simulink model "HevMmPowertrainController"  (R2020a)
settings: Solver=ode4  StartTime=0.0  StopTime=inf  FixedStep=.01  RelTol=1e-3  EnableMultiTasking=on
model workspace (MAT data in the model file):
  ChrgSOCHi = 80
  ChrgSOCLo = 70
  EngCltchOffTractiveForce = 3000
  EngCltchOffVehSpd = 70
  EngCltchOnTractiveForce = 2000
  EngCltchOnVehSpd = 80
  EngCltchOnWait = 5
  EngDriveRatio = 0.813008130081
  FricBrakeCmd = [0 0 12 24 36 48 60]
  FricBrakeCmdBpt = [0 0.1 0.2 0.4 0.6 0.8 1]
  MaxChrgPwr = 50000
  MaxRegenPwr = 10000
  MotGbRatio = 2.45
  Ndiff = 3.421
  Rm = 0.17778
  Ts = 0.01
  disk_abore = 0.05
  eng.pwr = [15052.6315789 19736.8421053 24421.0526316 29105.2631579 33789.4736842 38473.6842105 43157.8947368 47842.1052632 52526.3157895 57210.5263158 61894.7368421 66578.9473684 71263.1578947 75947.3684211 80631.5789474 85315.7894737 90000]
  eng.spd = [1448.84862461 1712.99052669 1980.33600187 2249.1155588 2517.55970613 2783.89895252 3046.3638066 3303.18477703 3552.59237246 3792.81710154 4022.08947291 4238.63999523 4440.69917715 4626.49752731 4794.26555436 4942.23376695 5068.63267374]
  eng.bsfc = [256.743221884 250.98807985 246.162934447 242.291845325 239.398872138 237.508074537 236.643512177 236.829244708 238.089331783 240.447833055 243.928808176 248.556316798 254.354418575 261.347173158 269.5586402 279.012879353 289.73395027]
  eng.trq = [99.2112225513 110.02568665 117.759751017 123.57514891 128.166058939 131.971967205 135.285068696 138.308475993 141.18967656 144.040766791 146.951280713 149.9967243 153.244568751 156.75874496 160.603298419 164.845657961 169.559869104]
  eng.idle = 1448.84862461
  eng.ff = [0.00107351698039 0.00137603113953 0.00166987721613 0.00195887997755 0.00224698941392 0.00253828073811 0.00283695438574 0.00314733601519 0.00347387650759 0.00382115196682 0.00419386371951 0.00459683831506 0.00503502752559 0.005513508346 0.00603748299394 0.00661227890981 0.00724334875674]
  eng.pwrin = [46556.889434 59676.4939829 72420.1762428 84953.8108807 97448.7032942 110081.589612 123034.636693 136495.442128 150657.034239 165717.872078 181881.845427 199358.274801 218361.911444 239112.937333 261836.965174 286765.038405 314133.631195]
  gen.max_trq = 247.580645161
  gen.max_pwr = 102.101761242
  gen.spd = [0 500 1000 1500 2000 2500 3000 3500 3938.11074919 4000 4500 5000 5500 6000 6500 7000 7500 8000 8500 9000 9500 10000 10500 11000 11500 12000 12500]
  gen.trq = [247.580645161 247.580645161 247.580645161 247.580645161 247.580645161 247.580645161 247.580645161 247.580645161 247.580645161 243.75 216.666666667 195 177.272727273 162.5 150 139.285714286 130 121.875 114.705882353 108.333333333 102.631578947 97.5 92.8571428571 88.6363636364 84.7826086957 81.25 78]
  gen.trq_cp = [243.75 216.666666667 195 177.272727273 162.5 150 139.285714286 130 121.875 114.705882353 108.333333333 102.631578947 97.5 92.8571428571 88.6363636364 84.7826086957 81.25 78]
  gen.J = 0.02
  gen.damp = 0.001
  gen.Tc = 0.02
  gen.map.spdindex = [0 1000 2000 3000 3857 4000 5000 6000 7000 8000 9000 10000 11000 12000 12584]
  gen.map.trqindex = [10 25 50 75 100 125 150 175 200 225 235.201612903]
  gen.map.eff = [84  90  90  90  90  90  90  90  90  90  90  90  90  90  90; 84  90  93  95  95  95  96  95  95  95  95  93  93  93  93; 84  90  93  95  95  95  96  95  96  95  95  95  95  93  93; 84  90  93  95  95  95  96  96  96  95  95  93  95  93  93; 84  90  93  95  95  95  96  96  96  95  95  93  93  93  93; 84  88  90  93  93  95  95  96  95  93  93  93  93  93  93; 84  88  90  90  90  93  95  95  93  93  93  93  93  93  93; 84  88  90  90  90  90  93  93  93  93  93  93  93  93  93; 84  84  88  90  90  90  90  93  93  93  93  93  93  93  93; 84  84  88  90  90  90  90  93  93  93  93  93  93  93  93; 84  84  88  90  90  90  90  93  93  93  93  93  93  93  93]
  gen.m = 20
  gen.Cp = 200
  mot.max_trq = 307
  mot.max_pwr = 124
  mot.spd = [0 500 1000 1500 2000 2500 3000 3500 3857.04487493 4000 4500 5000 5500 6000 6500 7000 7500 8000 8500 9000 9500 10000 10500 11000 11500 12000 12500]
  mot.trq = [307 307 307 307 307 307 307 307 307 296.028194151 263.136172579 236.822555321 215.29323211 197.352129434 182.171196401 169.158968086 157.881703547 148.014097075 139.307385483 131.568086289 124.643450169 118.41127766 112.772645391 107.646616055 102.9663284 98.676064717 94.7290221283]
  mot.trq_cp = [296.028194151 263.136172579 236.822555321 215.29323211 197.352129434 182.171196401 169.158968086 157.881703547 148.014097075 139.307385483 131.568086289 124.643450169 118.41127766 112.772645391 107.646616055 102.9663284 98.676064717 94.7290221283]
  mot.J = 0.02
  mot.damp = 0.0001
  mot.Tc = 0.0267
  mot.map.spdindex = [0 1000 2000 3000 3857 4000 5000 6000 7000 8000 9000 10000 11000 12000 12584]
  mot.map.trqindex = [10 25 50 75 100 125 150 175 200 225 250 275 300 307]
  mot.map.eff = [84  90  90  90  90  90  90  90  90  90  90  90  90  90  90; 84  90  93  95  95  95  96  95  95  95  95  93  93  93  93; 84  90  93  95  95  95  96  95  96  95  95  95  95  93  93; 84  90  93  95  95  95  96  96  96  95  95  95  95  93  93; 84  90  93  95  95  95  96  96  96  95  95  93  93  93  90; 84  88  90  93  93  95  95  96  95  95  95  93  93  93  90; 84  88  90  90  90  93  95  95  95  93  93  93  93  93  90; 84  88  90  90  90  90  93  93  93  93  93  93  93  93  90; 84  84  88  90  90  90  93  93  93  93  93  93  93  93  90; 84  84  88  90  90  90  90  93  93  93  93  93  93  93  90; 84  84  84  90  90  90  90  93  93  93  93  93  93  93  90; 84  84  84  88  90  90  90  93  93  93  93  93  93  93  90; 84  84  84  88  88  88  90  93  93  93  93  93  93  93  90; 84  84  84  88  88  88  90  93  93  93  93  93  93  93  90]
  mot.m = 30
  mot.Cp = 200
  mu_kinetic = 0.2
  num_pads = 2
values from neighbouring files (symbols this model uses):
  eng : value not decoded    [HevMmPowertrainControllerDD.sldd]
  mot = 307.0    [HevMmPowertrainControllerDD.sldd]
libraries: simulink x3, autolibutils x1
settings Model: ModifiedByFormat=The MathWorks, Inc.  Creator=The MathWorks, Inc.  LastModifiedBy=The MathWorks, Inc.
settings DataIOCC: ReturnWorkspaceOutputs=off
settings DebuggingCC: UnderspecifiedInitializationDetection=Classic  MergeDetectMultiDrivingBlocksExec=none  SFNoUnconditionalDefaultTransitionDiag=warning  ArithmeticOperatorsInVariantConditions=warning
settings SFSimCC: SimUseLocalCustomCode=off
settings RTWCC: RTWUseLocalCustomCode=off
settings CodeAppCC: StateflowObjectComments=on
settings GRTTargetCC: TargetLangStandard=C89/C90 (ANSI)
settings ConfigComp: CovMetricSettings=dsw  CovHtmlReporting=on  CovSaveCumulativeToWorkspaceVar=on  CovSaveSingleToWorkspaceVar=on  CovShowResultsExplorer=off  CovExternalEMLEnable=off

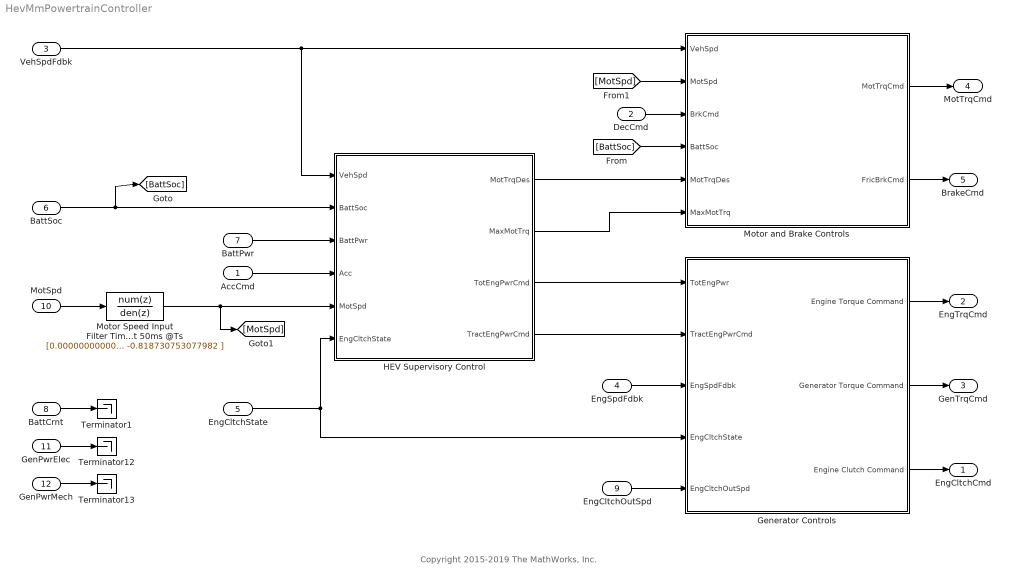
== system HevMmPowertrainController ==
  note: Copyright 2015-2019 The MathWorks, Inc.
  AccCmd : Inport
  DecCmd : Inport  Port=2  OutDataTypeStr=double
  VehSpdFdbk : Inport  Port=3
  EngSpdFdbk : Inport  Port=4
  EngCltchState : Inport  Port=5
  BattSoc : Inport  Port=6
  BattPwr : Inport  Port=7
  BattCrnt : Inport  Port=8
  EngCltchOutSpd : Inport  Port=9
  MotSpd : Inport  Port=10
  GenPwrElec : Inport  Port=11
  GenPwrMech : Inport  Port=12
  Generator Controls : Subsystem
  HEV Supervisory Control : Subsystem
  Motor Speed Input Filter Time Constant 50ms @Ts : DiscreteTransferFcn  Numerator=[0.000000000000000 0.181269246922018 ]  Denominator=[1.000000000000000 -0.818730753077982 ]  mask(DiscretizedDiscreteTransferFcn){}
      mask init:
      | %zoh
  Motor and Brake Controls : Subsystem
  Terminator1 : Terminator
  Terminator12 : Terminator
  Terminator13 : Terminator
  EngCltchCmd : Outport  VectorParamsAs1DForOutWhenUnconnected=off
  EngTrqCmd : Outport  Port=2  VectorParamsAs1DForOutWhenUnconnected=off
  GenTrqCmd : Outport  Port=3  VectorParamsAs1DForOutWhenUnconnected=off
  MotTrqCmd : Outport  Port=4  VectorParamsAs1DForOutWhenUnconnected=off
  BrakeCmd : Outport  Port=5  VectorParamsAs1DForOutWhenUnconnected=off
  wires:
  BattCrnt/1 -> Terminator1/1
  Motor and Brake Controls/1(MotTrqCmd) -> MotTrqCmd/1
  VehSpdFdbk/1 -> Motor and Brake Controls/1(VehSpd), HEV Supervisory Control/1(VehSpd)
  DecCmd/1 -> Motor and Brake Controls/3(BrkCmd)
  EngCltchState/1 -> HEV Supervisory Control/6(EngCltchState), Generator Controls/4(EngCltchState)
  HEV Supervisory Control/1(MotTrqDes) -> Motor and Brake Controls/5(MotTrqDes)
  Generator Controls/3(Engine Clutch Command) -> EngCltchCmd/1
  Motor and Brake Controls/2(FricBrkCmd) -> BrakeCmd/1
  [MotSpd] -> Motor and Brake Controls/2(MotSpd)
  EngCltchOutSpd/1 -> Generator Controls/5(EngCltchOutSpd)
  BattSoc/1 -> [BattSoc], HEV Supervisory Control/2(BattSoc)
  Motor Speed Input Filter Time Constant 50ms @Ts/1 -> [MotSpd], HEV Supervisory Control/5(MotSpd)
  [BattSoc] -> Motor and Brake Controls/4(BattSoc)
  Generator Controls/2(Generator Torque Command) -> GenTrqCmd/1
  EngSpdFdbk/1 -> Generator Controls/3(EngSpdFdbk)
  BattPwr/1 -> HEV Supervisory Control/3(BattPwr)
  AccCmd/1 -> HEV Supervisory Control/4(Acc)
  HEV Supervisory Control/3(TotEngPwrCmd) -> Generator Controls/1(TotEngPwr)
  Generator Controls/1(Engine Torque Command) -> EngTrqCmd/1
  HEV Supervisory Control/4(TractEngPwrCmd) -> Generator Controls/2(TractEngPwrCmd)
  GenPwrMech/1 -> Terminator13/1
  HEV Supervisory Control/2(MaxMotTrq) -> Motor and Brake Controls/6(MaxMotTrq)
  GenPwrElec/1 -> Terminator12/1
  MotSpd/1 -> Motor Speed Input Filter Time Constant 50ms @Ts/1

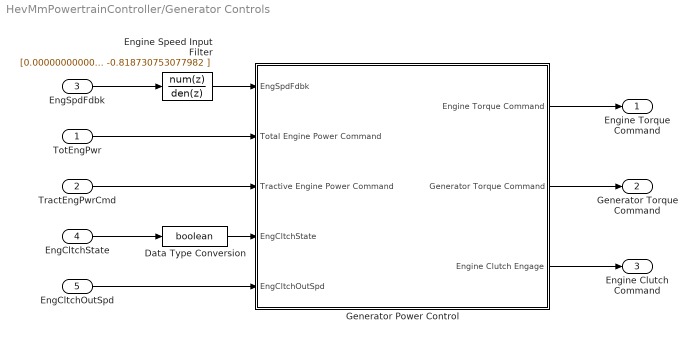
== system HevMmPowertrainController/Generator Controls ==
  TotEngPwr : Inport
  TractEngPwrCmd : Inport  Port=2
  EngSpdFdbk : Inport  Port=3
  EngCltchState : Inport  Port=4
  EngCltchOutSpd : Inport  Port=5
  Data Type Conversion : DataTypeConversion  OutDataTypeStr=boolean
  Engine Speed Input Filter : DiscreteTransferFcn  Numerator=[0.000000000000000 0.181269246922018 ]  Denominator=[1.000000000000000 -0.818730753077982 ]  mask(DiscretizedDiscreteTransferFcn){}
      mask init:
      | %zoh
  Generator Power Control : Subsystem
  Engine Torque Command : Outport  VectorParamsAs1DForOutWhenUnconnected=off
  Generator Torque Command : Outport  Port=2  VectorParamsAs1DForOutWhenUnconnected=off
  Engine Clutch Command : Outport  Port=3  VectorParamsAs1DForOutWhenUnconnected=off
  wires:
  EngSpdFdbk/1 -> Engine Speed Input Filter/1
  Generator Power Control/1(Engine Torque Command) -> Engine Torque Command/1
  Generator Power Control/2(Generator Torque Command) -> Generator Torque Command/1
  Engine Speed Input Filter/1 -> Generator Power Control/1(EngSpdFdbk)
  EngCltchOutSpd/1 -> Generator Power Control/5(EngCltchOutSpd)
  Generator Power Control/3(Engine Clutch Engage) -> Engine Clutch Command/1
  TractEngPwrCmd/1 -> Generator Power Control/3(Tractive Engine Power Command)
  EngCltchState/1 -> Data Type Conversion/1
  TotEngPwr/1 -> Generator Power Control/2(Total Engine Power Command)
  Data Type Conversion/1 -> Generator Power Control/4(EngCltchState)

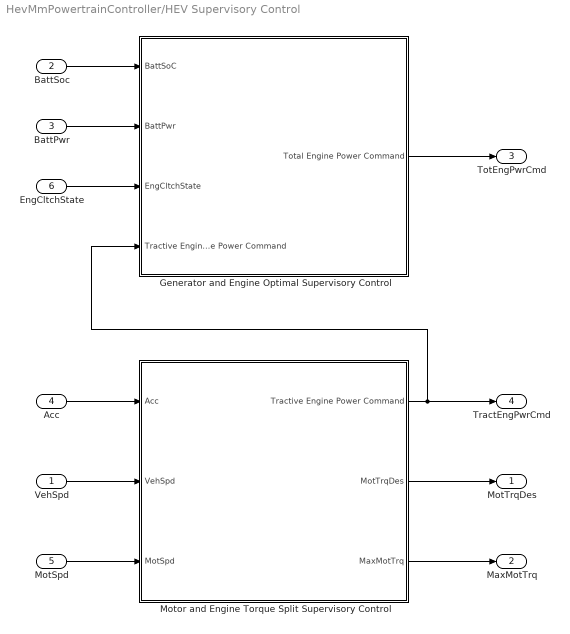
== system HevMmPowertrainController/HEV Supervisory Control ==
  VehSpd : Inport
  BattSoc : Inport  Port=2
  BattPwr : Inport  Port=3
  Acc : Inport  Port=4
  MotSpd : Inport  Port=5
  EngCltchState : Inport  Port=6
  Generator and Engine Optimal Supervisory Control : Subsystem
  Motor and Engine Torque Split Supervisory Control : Subsystem
  MotTrqDes : Outport  VectorParamsAs1DForOutWhenUnconnected=off
  MaxMotTrq : Outport  Port=2  VectorParamsAs1DForOutWhenUnconnected=off
  TotEngPwrCmd : Outport  Port=3  VectorParamsAs1DForOutWhenUnconnected=off
  TractEngPwrCmd : Outport  Port=4  VectorParamsAs1DForOutWhenUnconnected=off
  wires:
  Acc/1 -> Motor and Engine Torque Split Supervisory Control/1(Acc)
  VehSpd/1 -> Motor and Engine Torque Split Supervisory Control/2(VehSpd)
  MotSpd/1 -> Motor and Engine Torque Split Supervisory Control/3(MotSpd)
  Motor and Engine Torque Split Supervisory Control/2(MotTrqDes) -> MotTrqDes/1
  Motor and Engine Torque Split Supervisory Control/3(MaxMotTrq) -> MaxMotTrq/1
  Motor and Engine Torque Split Supervisory Control/1(Tractive Engine Power Command) -> Generator and Engine Optimal Supervisory Control/4(Tractive Engine Power Command), TractEngPwrCmd/1
  BattSoc/1 -> Generator and Engine Optimal Supervisory Control/1(BattSoC)
  BattPwr/1 -> Generator and Engine Optimal Supervisory Control/2(BattPwr)
  Generator and Engine Optimal Supervisory Control/1(Total Engine Power Command) -> TotEngPwrCmd/1
  EngCltchState/1 -> Generator and Engine Optimal Supervisory Control/3(EngCltchState)

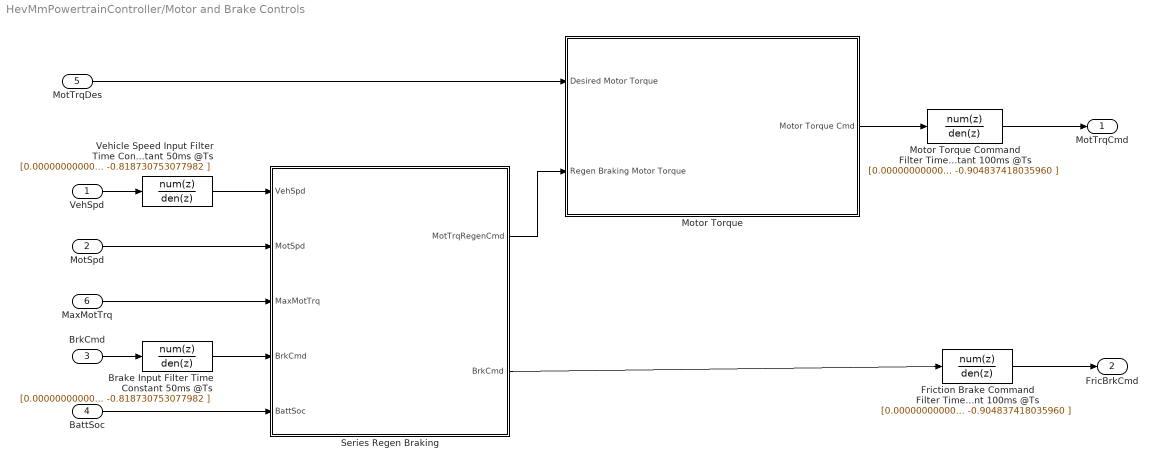
== system HevMmPowertrainController/Motor and Brake Controls ==
  VehSpd : Inport
  MotSpd : Inport  Port=2
  BrkCmd : Inport  Port=3
  BattSoc : Inport  Port=4
  MotTrqDes : Inport  Port=5
  MaxMotTrq : Inport  Port=6
  Brake Input Filter Time Constant 50ms @Ts : DiscreteTransferFcn  Numerator=[0.000000000000000 0.181269246922018 ]  Denominator=[1.000000000000000 -0.818730753077982 ]  mask(DiscretizedDiscreteTransferFcn){}
      mask init:
      | %zoh
  Friction Brake Command Filter Time constant 100ms @Ts : DiscreteTransferFcn  Numerator=[0.000000000000000 0.095162581964040 ]  Denominator=[1.000000000000000 -0.904837418035960 ]  mask(DiscretizedDiscreteTransferFcn){}
      mask init:
      | %zoh
  Motor Torque : Subsystem
  Motor Torque Command Filter Time constant 100ms @Ts : DiscreteTransferFcn  Numerator=[0.000000000000000 0.095162581964040 ]  Denominator=[1.000000000000000 -0.904837418035960 ]  mask(DiscretizedDiscreteTransferFcn){}
      mask init:
      | %zoh
  Series Regen Braking : Subsystem  VariantControl=0
  Vehicle Speed Input Filter Time Constant 50ms @Ts : DiscreteTransferFcn  Numerator=[0.000000000000000 0.181269246922018 ]  Denominator=[1.000000000000000 -0.818730753077982 ]  mask(DiscretizedDiscreteTransferFcn){}
      mask init:
      | %zoh
  MotTrqCmd : Outport  VectorParamsAs1DForOutWhenUnconnected=off
  FricBrkCmd : Outport  Port=2  VectorParamsAs1DForOutWhenUnconnected=off
  wires:
  VehSpd/1 -> Vehicle Speed Input Filter Time Constant 50ms @Ts/1
  Motor Torque/1(Motor Torque Cmd) -> Motor Torque Command Filter Time constant 100ms @Ts/1
  BrkCmd/1 -> Brake Input Filter Time Constant 50ms @Ts/1
  Series Regen Braking/1(" MotTrqRegenCmd") -> Motor Torque/2(Regen Braking Motor Torque)
  BattSoc/1 -> Series Regen Braking/5(BattSoc)
  MotTrqDes/1 -> Motor Torque/1(Desired Motor Torque)
  MotSpd/1 -> Series Regen Braking/2(MotSpd)
  Brake Input Filter Time Constant 50ms @Ts/1 -> Series Regen Braking/4(BrkCmd)
  Motor Torque Command Filter Time constant 100ms @Ts/1 -> MotTrqCmd/1
  Friction Brake Command Filter Time constant 100ms @Ts/1 -> FricBrkCmd/1
  Vehicle Speed Input Filter Time Constant 50ms @Ts/1 -> Series Regen Braking/1(VehSpd)
  MaxMotTrq/1 -> Series Regen Braking/3(MaxMotTrq)
  Series Regen Braking/2(" BrkCmd") -> Friction Brake Command Filter Time constant 100ms @Ts/1

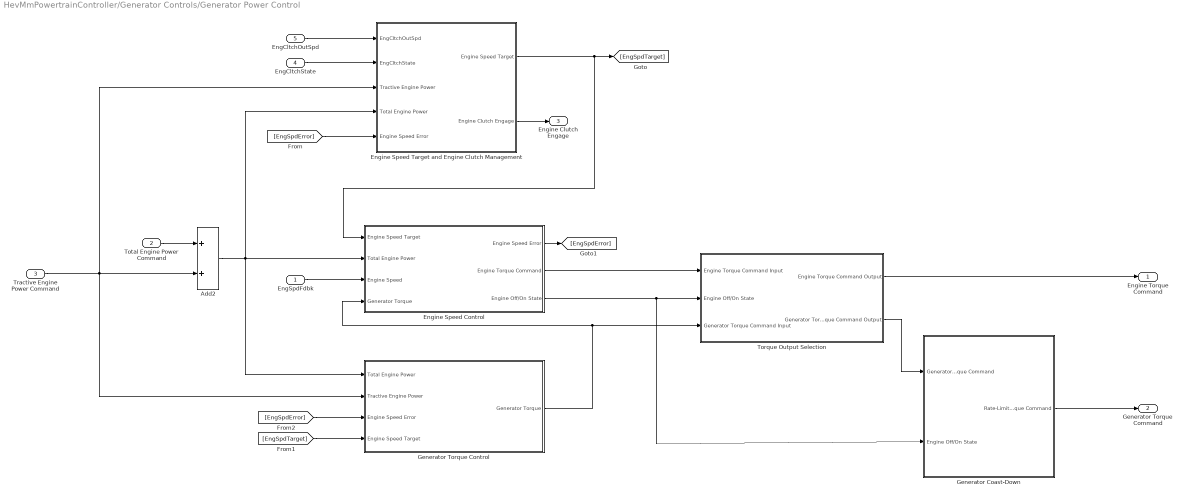
== system HevMmPowertrainController/Generator Controls/Generator Power Control ==
  EngSpdFdbk : Inport
  Total Engine Power Command : Inport  Port=2
  Tractive Engine Power Command : Inport  Port=3
  EngCltchState : Inport  Port=4
  EngCltchOutSpd : Inport  Port=5
  Add2 : Sum
  Engine Speed Control : Subsystem
  Engine Speed Target and Engine Clutch Management : Subsystem
  Generator Coast-Down : Subsystem
  Generator Torque Control : Subsystem
  Torque Output Selection : Subsystem
  Engine Torque Command : Outport  VectorParamsAs1DForOutWhenUnconnected=off
  Generator Torque Command : Outport  Port=2  VectorParamsAs1DForOutWhenUnconnected=off
  Engine Clutch Engage : Outport  Port=3  VectorParamsAs1DForOutWhenUnconnected=off
  wires:
  Add2/1 -> Engine Speed Target and Engine Clutch Management/4(Total Engine Power), Generator Torque Control/1(Total Engine Power), Engine Speed Control/2(Total Engine Power)
  Tractive Engine Power Command/1 -> Add2/2, Generator Torque Control/2(Tractive Engine Power), Engine Speed Target and Engine Clutch Management/3(Tractive Engine Power)
  Total Engine Power Command/1 -> Add2/1
  Engine Speed Target and Engine Clutch Management/1(Engine Speed Target) -> Engine Speed Control/1(Engine Speed Target), [EngSpdTarget]
  EngCltchOutSpd/1 -> Engine Speed Target and Engine Clutch Management/1(EngCltchOutSpd)
  EngCltchState/1 -> Engine Speed Target and Engine Clutch Management/2(EngCltchState)
  Engine Speed Target and Engine Clutch Management/2(Engine Clutch Engage) -> Engine Clutch Engage/1
  Engine Speed Control/3(Engine Off/On State) -> Generator Coast-Down/2(Engine Off/On State), Torque Output Selection/2(Engine Off/On State)
  Engine Speed Control/1(Engine Speed Error) -> [EngSpdError]
  EngSpdFdbk/1 -> Engine Speed Control/3(Engine Speed)
  [EngSpdTarget] -> Generator Torque Control/4(Engine Speed Target)
  Generator Torque Control/1(Generator Torque) -> Engine Speed Control/4(Generator Torque), Torque Output Selection/3(Generator Torque Command Input)
  [EngSpdError] -> Engine Speed Target and Engine Clutch Management/5(Engine Speed Error)
  [EngSpdError] -> Generator Torque Control/3(Engine Speed Error)
  Engine Speed Control/2(Engine Torque Command) -> Torque Output Selection/1(Engine Torque Command Input)
  Torque Output Selection/2(Generator Torque Command Output) -> Generator Coast-Down/1(Generator Torque Command)
  Torque Output Selection/1(Engine Torque Command Output) -> Engine Torque Command/1
  Generator Coast-Down/1(Rate-Limited Generator Torque Command) -> Generator Torque Command/1

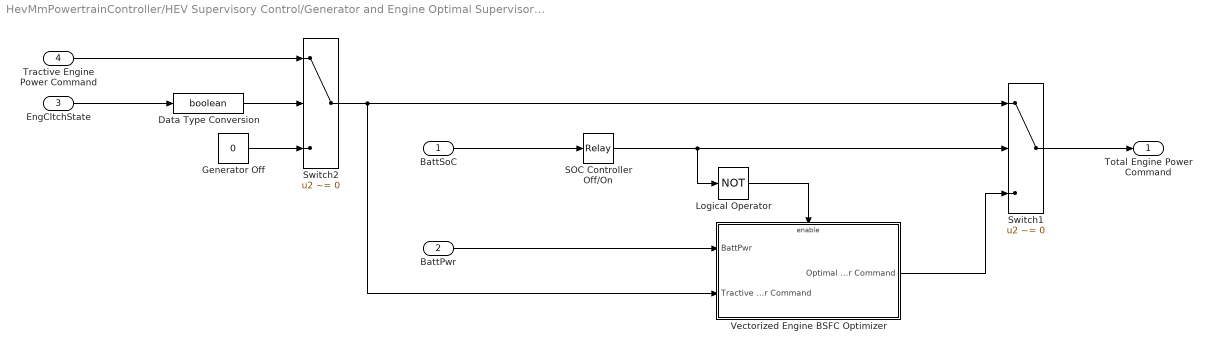
== system HevMmPowertrainController/HEV Supervisory Control/Generator and Engine Optimal Supervisory Control ==
  BattSoC : Inport
  BattPwr : Inport  Port=2
  EngCltchState : Inport  Port=3
  Tractive Engine Power Command : Inport  Port=4
  Data Type Conversion : DataTypeConversion  OutDataTypeStr=boolean
  Generator Off : Constant  Value=0
  Logical Operator : Logic  Operator=NOT  AllPortsSameDT=off  OutDataTypeStr=boolean
  SOC Controller Off/On : Relay  OnSwitchValue=ChrgSOCHi  OffSwitchValue=ChrgSOCLo  OnOutputValue=true  OffOutputValue=false
  Switch1 : Switch  Criteria=u2 ~= 0
  Switch2 : Switch  Criteria=u2 ~= 0
  Vectorized Engine BSFC Optimizer : Subsystem
  Total Engine Power Command : Outport  VectorParamsAs1DForOutWhenUnconnected=off
  wires:
  Switch1/1 -> Total Engine Power Command/1
  BattSoC/1 -> SOC Controller Off/On/1
  SOC Controller Off/On/1 -> Logical Operator/1, Switch1/2
  Vectorized Engine BSFC Optimizer/1(Optimal Engine Power Command) -> Switch1/3
  Logical Operator/1 -> Vectorized Engine BSFC Optimizer/Enable
  Switch2/1 -> Vectorized Engine BSFC Optimizer/2(Tractive Engine Power Command), Switch1/1
  BattPwr/1 -> Vectorized Engine BSFC Optimizer/1(BattPwr)
  Tractive Engine Power Command/1 -> Switch2/1
  EngCltchState/1 -> Data Type Conversion/1
  Generator Off/1 -> Switch2/3
  Data Type Conversion/1 -> Switch2/2

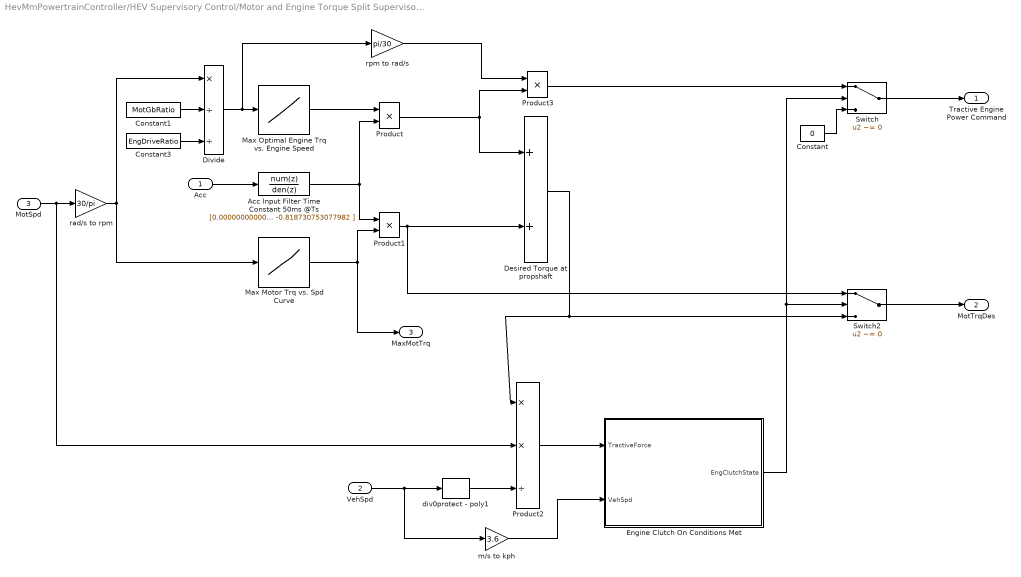
== system HevMmPowertrainController/HEV Supervisory Control/Motor and Engine Torque Split Supervisory Control ==
  Acc : Inport
  VehSpd : Inport  Port=2
  MotSpd : Inport  Port=3
  Acc Input Filter Time Constant 50ms @Ts : DiscreteTransferFcn  Numerator=[0.000000000000000 0.181269246922018 ]  Denominator=[1.000000000000000 -0.818730753077982 ]  mask(DiscretizedDiscreteTransferFcn){}
      mask init:
      | %zoh
  Constant : Constant  Value=0
  Constant1 : Constant  Value=MotGbRatio
  Constant3 : Constant  Value=EngDriveRatio
  Desired Torque at propshaft : Sum
  Divide : Product  Inputs=*//
  Engine Clutch On Conditions Met : Stateflow chart  TreatAsAtomicUnit=on
  Max Motor Trq vs. Spd Curve : Lookup_n-D  NumberOfTableDimensions=1  BreakpointsForDimension1=mot.spd  Table=mot.trq  ExtrapMethod=Clip  UseLastTableValue=on  InternalRulePriority=Speed  OutDataTypeStr=Inherit: Inherit from 'Table data'  RndMeth=Simplest  InputSameDT=on
  Max Optimal Engine Trq vs. Engine Speed : Lookup_n-D  NumberOfTableDimensions=1  BreakpointsForDimension1=eng.spd  Table=eng.trq  ExtrapMethod=Clip  UseLastTableValue=on  InternalRulePriority=Speed  OutDataTypeStr=Inherit: Inherit from 'Table data'  RndMeth=Simplest  InputSameDT=on
  Product : Product
  Product1 : Product
  Product2 : Product  Inputs=**/
  Product3 : Product
  Switch : Switch  Criteria=u2 ~= 0  Threshold=0.5
  Switch2 : Switch  Criteria=u2 ~= 0  Threshold=0.5
  div0protect - poly1 : autolibutils/div0protect - poly  thresh=1e-6  aMode=aMode
      settings: SourceProductBaseCode=PW,MT,VE,VP
  m/s to kph : Gain  Gain=3.6
  rad/s to rpm : Gain  Gain=30/pi
  rpm to rad/s : Gain  Gain=pi/30
  Tractive Engine Power Command : Outport  VectorParamsAs1DForOutWhenUnconnected=off
  MotTrqDes : Outport  Port=2  VectorParamsAs1DForOutWhenUnconnected=off
  MaxMotTrq : Outport  Port=3  VectorParamsAs1DForOutWhenUnconnected=off
  wires:
  Acc Input Filter Time Constant 50ms @Ts/1 -> Product1/1, Product/2
  Product1/1 -> Switch2/1, Desired Torque at propshaft/2
  Switch2/1 -> MotTrqDes/1
  Constant/1 -> Switch/3
  Switch/1 -> Tractive Engine Power Command/1
  rad/s to rpm/1 -> Divide/1, Max Motor Trq vs. Spd Curve/1
  Max Motor Trq vs. Spd Curve/1 -> MaxMotTrq/1, Product1/2
  Max Optimal Engine Trq vs. Engine Speed/1 -> Product/1
  Divide/1 -> rpm to rad/s/1, Max Optimal Engine Trq vs. Engine Speed/1
  Constant1/1 -> Divide/2
  Acc/1 -> Acc Input Filter Time Constant 50ms @Ts/1
  Constant3/1 -> Divide/3
  Desired Torque at propshaft/1 -> Product2/1, Switch2/3
  VehSpd/1 -> m/s to kph/1, div0protect - poly1/1
  MotSpd/1 -> Product2/2, rad/s to rpm/1
  div0protect - poly1/1 -> Product2/3
  m/s to kph/1 -> Engine Clutch On Conditions Met/2(VehSpd)
  Engine Clutch On Conditions Met/1(EngClutchState) -> Switch2/2, Switch/2
  Product2/1 -> Engine Clutch On Conditions Met/1(TractiveForce)
  Product/1 -> Product3/2, Desired Torque at propshaft/1
  rpm to rad/s/1 -> Product3/1
  Product3/1 -> Switch/1

== system HevMmPowertrainController/Motor and Brake Controls/Motor Torque ==
  Desired Motor Torque : Inport
  Regen Braking Motor Torque : Inport  Port=2
  Accel Decel Switch : Switch  Criteria=u2 ~= 0
  Compare To Constant : simulink/Logic and Bit Operations/Compare To Constant  relop=>  const=1e-6  OutDataTypeStr=boolean
  Motor Torque Cmd : Outport  VectorParamsAs1DForOutWhenUnconnected=off
  wires:
  Regen Braking Motor Torque/1 -> Accel Decel Switch/3
  Accel Decel Switch/1 -> Motor Torque Cmd/1
  Desired Motor Torque/1 -> Compare To Constant/1, Accel Decel Switch/1
  Compare To Constant/1 -> Accel Decel Switch/2

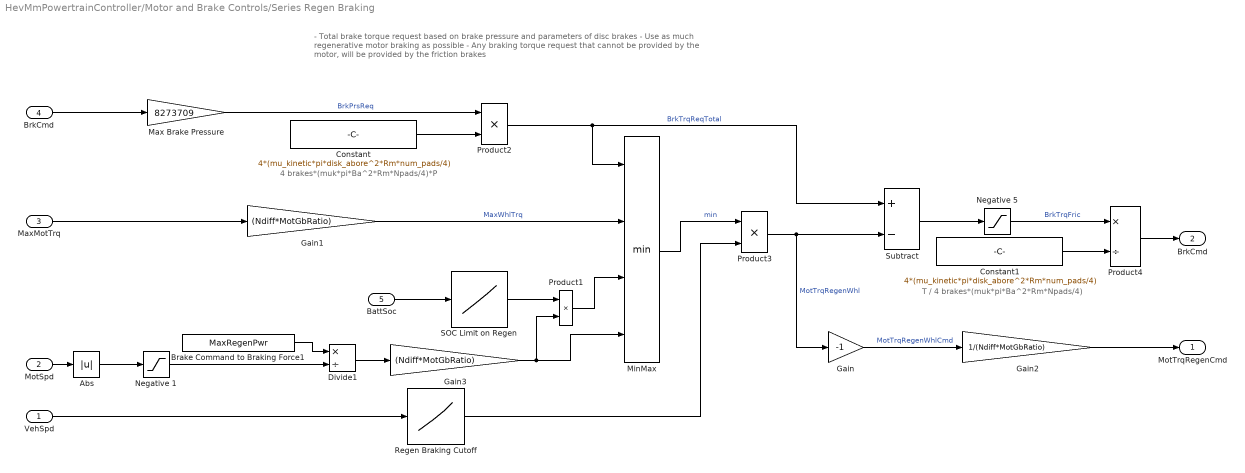
== system HevMmPowertrainController/Motor and Brake Controls/Series Regen Braking ==
  note: - Total brake torque request based on brake pressure and parameters of disc brakes
      | - Use as much regenerative motor braking as possible
      | -  Any braking torque request that cannot be provided by the motor, will be provided by the friction brakes
  note: T / 4 brakes*(muk*pi*Ba^2*Rm*Npads/4)
  note: 4 brakes*(muk*pi*Ba^2*Rm*Npads/4)*P
  VehSpd : Inport
  MotSpd : Inport  Port=2
  MaxMotTrq : Inport  Port=3
  BrkCmd : Inport  Port=4
  BattSoc : Inport  Port=5
  Abs : Abs  ZeroCross=off
  Brake Command to Braking Force1 : Constant  Value=MaxRegenPwr
  Constant : Constant  Value=4*(mu_kinetic*pi*disk_abore^2*Rm*num_pads/4)
  Constant1 : Constant  Value=4*(mu_kinetic*pi*disk_abore^2*Rm*num_pads/4)
  Divide1 : Product  Inputs=*/
  Gain : Gain  Gain=-1
  Gain1 : Gain  Gain=(Ndiff*MotGbRatio)
  Gain2 : Gain  Gain=1/(Ndiff*MotGbRatio)
  Gain3 : Gain  Gain=(Ndiff*MotGbRatio)
  Max Brake Pressure : Gain  Gain=8273709
  MinMax : MinMax  Inputs=4
  Negative 1 : Saturate  UpperLimit=inf  LowerLimit=1
  Negative 5 : Saturate  UpperLimit=inf  LowerLimit=0
  Product1 : Product
  Product2 : Product
  Product3 : Product
  Product4 : Product  Inputs=*/
  Regen Braking Cutoff : Lookup_n-D  NumberOfTableDimensions=1  BreakpointsForDimension1=[0.5 1]  Table=[0 1]  ExtrapMethod=Clip  InternalRulePriority=Speed  RndMeth=Simplest  InputSameDT=on
  SOC Limit on Regen : Lookup_n-D  NumberOfTableDimensions=1  BreakpointsForDimension1=[80 90]  Table=[1 0]  ExtrapMethod=Clip  InternalRulePriority=Speed  RndMeth=Simplest  InputSameDT=on
  Subtract : Sum  Inputs=+-
  " MotTrqRegenCmd" : Outport  VectorParamsAs1DForOutWhenUnconnected=off
  " BrkCmd" : Outport  Port=2  VectorParamsAs1DForOutWhenUnconnected=off
  wires:
  Product3/1 -> Gain/1, Subtract/2  "MotTrqRegenWhl"
  Product4/1 -> " BrkCmd"/1
  Constant1/1 -> Product4/2
  Constant/1 -> Product2/2
  BrkCmd/1 -> Max Brake Pressure/1
  MaxMotTrq/1 -> Gain1/1
  Product2/1 -> MinMax/1, Subtract/1  "BrkTrqReqTotal"
  MinMax/1 -> Product3/1  "min"
  Subtract/1 -> Negative 5/1
  Negative 5/1 -> Product4/1  "BrkTrqFric"
  Gain/1 -> Gain2/1  "MotTrqRegenWhlCmd"
  Gain1/1 -> MinMax/2  "MaxWhlTrq"
  Max Brake Pressure/1 -> Product2/1  "BrkPrsReq"
  VehSpd/1 -> Regen Braking Cutoff/1
  Regen Braking Cutoff/1 -> Product3/2
  Gain2/1 -> " MotTrqRegenCmd"/1
  Product1/1 -> MinMax/3
  MotSpd/1 -> Abs/1
  BattSoc/1 -> SOC Limit on Regen/1
  SOC Limit on Regen/1 -> Product1/1
  Divide1/1 -> Gain3/1
  Brake Command to Braking Force1/1 -> Divide1/1
  Abs/1 -> Negative 1/1
  Negative 1/1 -> Divide1/2
  Gain3/1 -> Product1/2, MinMax/4

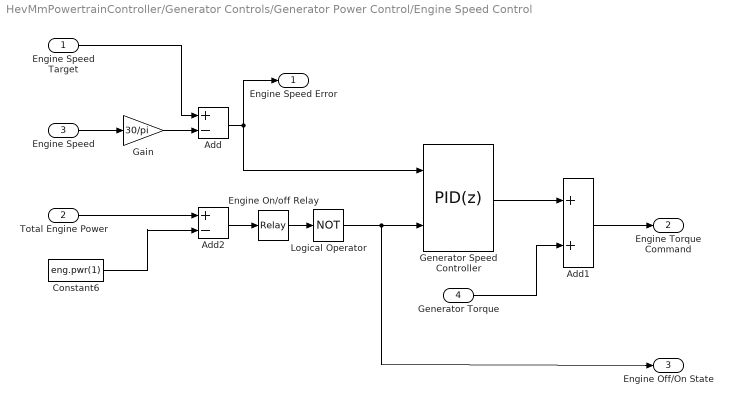
== system HevMmPowertrainController/Generator Controls/Generator Power Control/Engine Speed Control ==
  Engine Speed Target : Inport
  Total Engine Power : Inport  Port=2
  Engine Speed : Inport  Port=3
  Generator Torque : Inport  Port=4
  Add : Sum  Inputs=+-
  Add1 : Sum
  Add2 : Sum  Inputs=+-
  Constant6 : Constant  Value=eng.pwr(1)
  Engine On/off Relay : Relay  OnSwitchValue=1000  OffSwitchValue=0  OnOutputValue=true  OffOutputValue=false
  Gain : Gain  Gain=30/pi
  Generator Speed Controller : simulink/Continuous/PID Controller  Controller=PID  Form=Parallel  TimeDomain=Discrete-time  UseExternalTs=off  SampleTime=-1  IntegratorMethod=Forward Euler  FilterMethod=Forward Euler  ControllerParametersSource=internal  P=0.05  I=0.015  D=0  UseFilter=off  N=100  TunerSelectOption=Transfer Function Based (PID Tuner App)  InitialConditionSource=internal  InitialConditionForIntegrator=0  InitialConditionForFilter=0  DifferentiatorICPrevScaledInput=0  ExternalReset=level  TrackingMode=off  Kt=1  LimitOutput=on  UpperSaturationLimit=eng.trq(end)  LowerSaturationLimit=0  LinearizeAsGain=off  AntiWindupMode=clamping  Kb=1  POutMin=[]  POutMax=[]  IOutMin=[]  IOutMax=[]  DOutMin=[]  DOutMax=[]  NOutMin=[]  NOutMax=[]  SumOutMin=[]  SumOutMax=[]  SaturationOutMin=[]  SaturationOutMax=[]  PParamMin=[]  PParamMax=[]  IParamMin=[]  IParamMax=[]  DParamMin=[]  DParamMax=[]  NParamMin=[]  NParamMax=[]  KbParamMin=[]  KbParamMax=[]  KtParamMin=[]  KtParamMax=[]  KbOutMin=[]  KbOutMax=[]  KtOutMin=[]  KtOutMax=[]  IntegratorOutMin=[]  IntegratorOutMax=[]  FilterOutMin=[]  FilterOutMax=[]  SumI1OutMin=[]  SumI1OutMax=[]  SumI2OutMin=[]  SumI2OutMax=[]  SumI3OutMin=[]  SumI3OutMax=[]  SumI4OutMin=[]  SumI4OutMax=[]  SumDOutMin=[]  SumDOutMax=[]  DifferentiatorOutMin=[]  DifferentiatorOutMax=[]  FilterDiffOutCoefMin=[]  FilterDiffOutCoefMax=[]  ReciprocalOutMin=[]  ReciprocalOutMax=[]  SumDenOutMin=[]  SumDenOutMax=[]  SumNumOutMin=[]  SumNumOutMax=[]  DivideOutMin=[]  DivideOutMax=[]  UdiffTsProdOutMin=[]  UdiffTsProdOutMax=[]  NTsProdOutMin=[]  NTsProdOutMax=[]  UintegralTsProdOutMin=[]  UintegralTsProdOutMax=[]  UngainTsProdOutMin=[]  UngainTsProdOutMax=[]  IntegratorContinuousStateAttributes=''  IntegratorStateMustResolveToSignalObject=off  IntegratorRTWStateStorageClass=Auto  FilterContinuousStateAttributes=''  FilterStateMustResolveToSignalObject=off  FilterRTWStateStorageClass=Auto  ParallelPVariant=InternalParameters  IdealPVariant=Disabled  IVariant=InternalParameters  DVariant=InternalParameters  IntegratorVariant=Discrete  SatVariant=Enabled  AWVariant=DiscClampingParallel  PCopyVariant=Disabled  TRVariant=Disabled  FdbkBlocksVariant=Forward  IdealPFdbkVariant=Disabled  SatFdbkVariant=Disabled  DerivativeFilterVariant=Differentiator  NVariant=Passthrough  NCopyVariant=Disabled_SignalSpec  FilterICVariant=InternalICsDifferentiator  IntegratorICVariant=InternalICs  ExternalResetVariant=ExternalReset  TRSumVariant=Passthrough  SumFdbkVariant=Disabled  SumVariant=Sum_PID  TsampFilterVariant=InternalTs  TsampNgainVariant=Passthrough  TsampIntegralVariant=Passthrough
  Logical Operator : Logic  Operator=NOT  AllPortsSameDT=off  OutDataTypeStr=boolean
  Engine Speed Error : Outport  VectorParamsAs1DForOutWhenUnconnected=off
  Engine Torque Command : Outport  Port=2  VectorParamsAs1DForOutWhenUnconnected=off
  Engine Off/On State : Outport  Port=3  VectorParamsAs1DForOutWhenUnconnected=off
  wires:
  Total Engine Power/1 -> Add2/1
  Generator Torque/1 -> Add1/2
  Add/1 -> Generator Speed Controller/1, Engine Speed Error/1
  Engine Speed Target/1 -> Add/1
  Gain/1 -> Add/2
  Add1/1 -> Engine Torque Command/1
  Engine Speed/1 -> Gain/1
  Constant6/1 -> Add2/2
  Generator Speed Controller/1 -> Add1/1
  Logical Operator/1 -> Generator Speed Controller/2, Engine Off/On State/1
  Add2/1 -> Engine On/off Relay/1
  Engine On/off Relay/1 -> Logical Operator/1

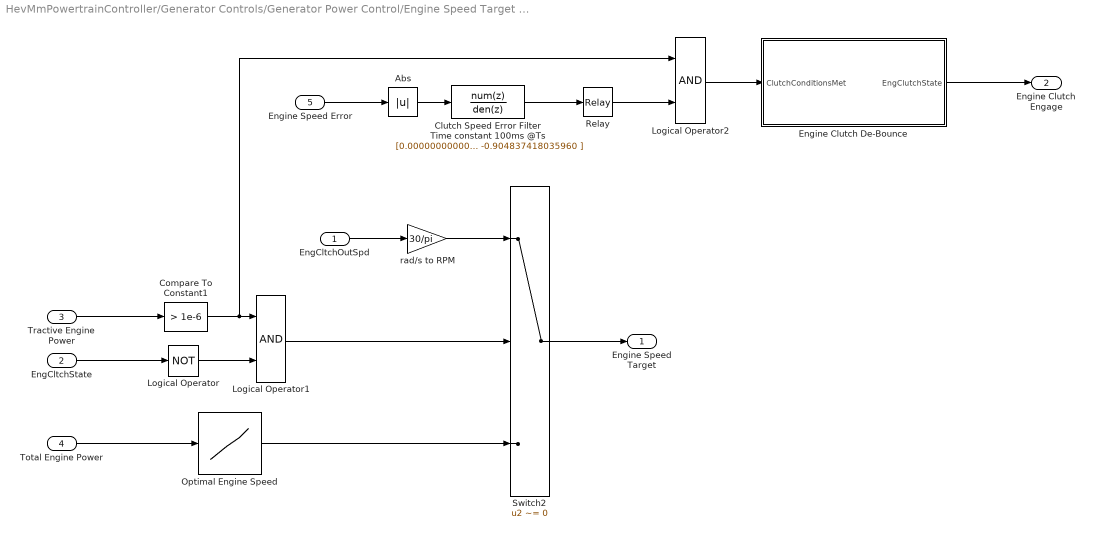
== system HevMmPowertrainController/Generator Controls/Generator Power Control/Engine Speed Target and Engine Clutch Management ==
  EngCltchOutSpd : Inport
  EngCltchState : Inport  Port=2
  Tractive Engine Power : Inport  Port=3
  Total Engine Power : Inport  Port=4
  Engine Speed Error : Inport  Port=5
  Abs : Abs
  Clutch Speed Error Filter Time constant 100ms @Ts : DiscreteTransferFcn  Numerator=[0.000000000000000 0.095162581964040 ]  Denominator=[1.000000000000000 -0.904837418035960 ]  mask(DiscretizedDiscreteTransferFcn){}
      mask init:
      | %zoh
  Compare To Constant1 : simulink/Logic and Bit Operations/Compare To Constant  relop=>  const=1e-6  OutDataTypeStr=boolean
  Engine Clutch De-Bounce : Stateflow chart  TreatAsAtomicUnit=on
  Logical Operator : Logic  Operator=NOT  AllPortsSameDT=off  OutDataTypeStr=boolean
  Logical Operator1 : Logic  AllPortsSameDT=off  OutDataTypeStr=boolean
  Logical Operator2 : Logic  AllPortsSameDT=off  OutDataTypeStr=boolean
  Optimal Engine Speed : Lookup_n-D  NumberOfTableDimensions=1  BreakpointsForDimension1=eng.pwr  Table=eng.spd  ExtrapMethod=Clip  InternalRulePriority=Speed  RndMeth=Simplest  InputSameDT=on
  Relay : Relay  OnSwitchValue=150  OffSwitchValue=100  OnOutputValue=false  OffOutputValue=true
  Switch2 : Switch  Criteria=u2 ~= 0
  rad/s to RPM : Gain  Gain=30/pi
  Engine Speed Target : Outport  VectorParamsAs1DForOutWhenUnconnected=off
  Engine Clutch Engage : Outport  Port=2  VectorParamsAs1DForOutWhenUnconnected=off
  wires:
  Switch2/1 -> Engine Speed Target/1
  Logical Operator1/1 -> Switch2/2
  Optimal Engine Speed/1 -> Switch2/3
  EngCltchState/1 -> Logical Operator/1
  Logical Operator/1 -> Logical Operator1/2
  EngCltchOutSpd/1 -> rad/s to RPM/1
  Total Engine Power/1 -> Optimal Engine Speed/1
  Compare To Constant1/1 -> Logical Operator2/1, Logical Operator1/1
  Abs/1 -> Clutch Speed Error Filter Time constant 100ms @Ts/1
  Clutch Speed Error Filter Time constant 100ms @Ts/1 -> Relay/1
  Relay/1 -> Logical Operator2/2
  Logical Operator2/1 -> Engine Clutch De-Bounce/1(ClutchConditionsMet)
  Engine Speed Error/1 -> Abs/1
  rad/s to RPM/1 -> Switch2/1
  Engine Clutch De-Bounce/1(EngClutchState) -> Engine Clutch Engage/1
  Tractive Engine Power/1 -> Compare To Constant1/1

== system HevMmPowertrainController/Generator Controls/Generator Power Control/Generator Coast-Down ==
  Generator Torque Command : Inport
  Engine Off/On State : Inport  Port=2
  Generator Coast-Down Rate Limit : RateLimiter  RisingSlewLimit=100  FallingSlewLimit=-Inf  SampleTimeMode=inherited
  Switch1 : Switch  Criteria=u2 ~= 0
  Rate-Limited Generator Torque Command : Outport  VectorParamsAs1DForOutWhenUnconnected=off
  wires:
  Switch1/1 -> Rate-Limited Generator Torque Command/1
  Generator Torque Command/1 -> Switch1/3, Generator Coast-Down Rate Limit/1
  Generator Coast-Down Rate Limit/1 -> Switch1/1
  Engine Off/On State/1 -> Switch1/2

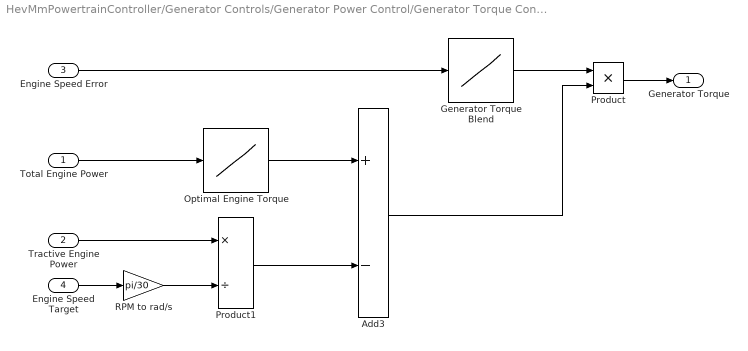
== system HevMmPowertrainController/Generator Controls/Generator Power Control/Generator Torque Control ==
  Total Engine Power : Inport
  Tractive Engine Power : Inport  Port=2
  Engine Speed Error : Inport  Port=3
  Engine Speed Target : Inport  Port=4
  Add3 : Sum  Inputs=+-
  Generator Torque Blend : Lookup_n-D  NumberOfTableDimensions=1  BreakpointsForDimension1=[0 200]  Table=[1 0]  ExtrapMethod=Clip  InternalRulePriority=Speed  RndMeth=Simplest  InputSameDT=on
  Optimal Engine Torque : Lookup_n-D  NumberOfTableDimensions=1  BreakpointsForDimension1=eng.pwr  Table=eng.trq  ExtrapMethod=Clip  InternalRulePriority=Speed  RndMeth=Simplest  InputSameDT=on
  Product : Product
  Product1 : Product  Inputs=*/
  RPM to rad/s : Gain  Gain=pi/30
  Generator Torque : Outport  VectorParamsAs1DForOutWhenUnconnected=off
  wires:
  Add3/1 -> Product/2
  Optimal Engine Torque/1 -> Add3/1
  Product/1 -> Generator Torque/1
  Generator Torque Blend/1 -> Product/1
  RPM to rad/s/1 -> Product1/2
  Product1/1 -> Add3/2
  Engine Speed Target/1 -> RPM to rad/s/1
  Total Engine Power/1 -> Optimal Engine Torque/1
  Tractive Engine Power/1 -> Product1/1
  Engine Speed Error/1 -> Generator Torque Blend/1

== system HevMmPowertrainController/Generator Controls/Generator Power Control/Torque Output Selection ==
  Engine Torque Command Input : Inport
  Engine Off/On State : Inport  Port=2
  Generator Torque Command Input : Inport  Port=3
  Constant : Constant  Value=[0 0]
  Demux : Demux  Outputs=2
  Gain1 : Gain  Gain=-1
  Mux : Mux  Inputs=2
  Switch : Switch  Criteria=u2 ~= 0
  Engine Torque Command Output : Outport  VectorParamsAs1DForOutWhenUnconnected=off
  Generator Torque Command Output : Outport  Port=2  VectorParamsAs1DForOutWhenUnconnected=off
  wires:
  Engine Torque Command Input/1 -> Mux/1
  Gain1/1 -> Mux/2
  Mux/1 -> Switch/3
  Demux/1 -> Engine Torque Command Output/1
  Constant/1 -> Switch/1
  Switch/1 -> Demux/1
  Generator Torque Command Input/1 -> Gain1/1
  Engine Off/On State/1 -> Switch/2
  Demux/2 -> Generator Torque Command Output/1

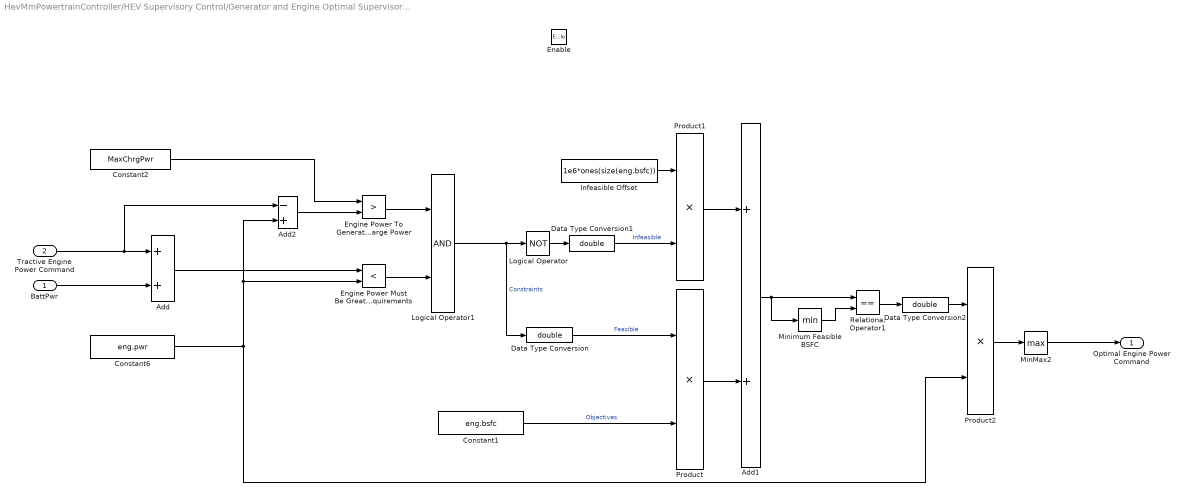
== system HevMmPowertrainController/HEV Supervisory Control/Generator and Engine Optimal Supervisory Control/Vectorized Engine BSFC Optimizer ==
  BattPwr : Inport
  Tractive Engine Power Command : Inport  Port=2
  Enable : EnablePort
  Add : Sum
  Add1 : Sum
  Add2 : Sum  Inputs=-+
  Constant1 : Constant  Value=eng.bsfc
  Constant2 : Constant  Value=MaxChrgPwr
  Constant6 : Constant  Value=eng.pwr
  Data Type Conversion : DataTypeConversion  OutDataTypeStr=double
  Data Type Conversion1 : DataTypeConversion  OutDataTypeStr=double
  Data Type Conversion2 : DataTypeConversion  OutDataTypeStr=double
  Engine Power Must Be Greater Than Tractive Power and Battery Draw Requirements : RelationalOperator  Operator=<  OutDataTypeStr=boolean  RndMeth=Simplest
  Engine Power To Generator Must Be Less Than Max Allowed Charge Power : RelationalOperator  Operator=>  OutDataTypeStr=boolean  RndMeth=Simplest
  Infeasible Offset : Constant  Value=1e6*ones(size(eng.bsfc))
  Logical Operator : Logic  Operator=NOT  AllPortsSameDT=off  OutDataTypeStr=boolean
  Logical Operator1 : Logic  AllPortsSameDT=off  OutDataTypeStr=boolean
  MinMax2 : MinMax  Function=max
  Minimum Feasible BSFC : MinMax
  Product : Product
  Product1 : Product
  Product2 : Product
  Relational Operator1 : RelationalOperator  Operator===  OutDataTypeStr=boolean  RndMeth=Simplest
  Optimal Engine Power Command : Outport  VectorParamsAs1DForOutWhenUnconnected=off
  wires:
  Constant1/1 -> Product/2  "Objectives"
  Data Type Conversion/1 -> Product/1  "Feasible"
  Product1/1 -> Add1/1
  MinMax2/1 -> Optimal Engine Power Command/1
  Infeasible Offset/1 -> Product1/1
  Data Type Conversion2/1 -> Product2/1
  Constant6/1 -> Product2/2, Engine Power Must Be Greater Than Tractive Power and Battery Draw Requirements/2, Add2/2
  Product2/1 -> MinMax2/1
  Data Type Conversion1/1 -> Product1/2  "Infeasible"
  Logical Operator/1 -> Data Type Conversion1/1
  Product/1 -> Add1/2
  Add1/1 -> Relational Operator1/1, Minimum Feasible BSFC/1
  Minimum Feasible BSFC/1 -> Relational Operator1/2
  Logical Operator1/1 -> Data Type Conversion/1, Logical Operator/1  "Constraints"
  Relational Operator1/1 -> Data Type Conversion2/1
  Add/1 -> Engine Power Must Be Greater Than Tractive Power and Battery Draw Requirements/1
  Constant2/1 -> Engine Power To Generator Must Be Less Than Max Allowed Charge Power/1
  Engine Power To Generator Must Be Less Than Max Allowed Charge Power/1 -> Logical Operator1/1
  Engine Power Must Be Greater Than Tractive Power and Battery Draw Requirements/1 -> Logical Operator1/2
  BattPwr/1 -> Add/2
  Tractive Engine Power Command/1 -> Add2/1, Add/1
  Add2/1 -> Engine Power To Generator Must Be Less Than Max Allowed Charge Power/2

== stateflow chart HevMmPowertrainController/Generator Controls/Generator Power Control/Engine Speed Target and Engine Clutch Management/Engine Clutch De-Bounce ==
  state ClutchOff
    en:
    EngClutchState=false;
  state ClutchOn
    en:
    OnWait=0.;
    EngClutchState=true;
    du:
    OnWait=OnWait+Ts;
  state ClutchHold
  (default) -> ClutchOff
  ClutchOff -> ClutchOn : [ClutchConditionsMet]
  ClutchHold -> ClutchOff : [~ClutchConditionsMet]
  ClutchOn -> ClutchHold : [OnWait>EngCltchOnWait]
  data: ClutchConditionsMet input; EngClutchState output; Ts parameter; EngCltchOnWait parameter; OnWait local

== stateflow chart HevMmPowertrainController/HEV Supervisory Control/Motor and Engine Torque Split Supervisory Control/Engine Clutch On Conditions Met ==
  state ClutchOff
    en:
    EngClutchState=false;
  state ClutchWait
    en:
    OnWait=0.;
    du:
    OnWait=OnWait+Ts;
  state ClutchOn
    en:
    EngClutchState=true;
  (default) -> ClutchOff
  ClutchOff -> ClutchWait : [(TractiveForce<EngCltchOnTractiveForce)&&...
      | (VehSpd>EngCltchOnVehSpd)]
  ClutchWait -> ClutchOff [order 1] : [(TractiveForce>EngCltchOffTractiveForce)||...
      | (VehSpd<EngCltchOffVehSpd)]
  ClutchOn -> ClutchOff : [(TractiveForce>EngCltchOffTractiveForce)||...
      | (VehSpd<EngCltchOffVehSpd)]
  ClutchWait -> ClutchOn [order 2] : [OnWait>EngCltchOnWait]
  data: TractiveForce input; VehSpd input; EngClutchState output; EngCltchOffVehSpd parameter; EngCltchOffTractiveForce parameter; EngCltchOnVehSpd parameter; EngCltchOnTractiveForce parameter; Ts parameter; EngCltchOnWait parameter; OnWait local
